simulink model "BSCU_Duration"  (Simulink 8.7)
settings: Solver=VariableStepAuto  StartTime=0.0  StopTime=10.0  RelTol=1e-3
settings Model: Creator=bourbouh  LastModifiedBy=bourbouh
settings DataIOCC: LimitDataPoints=off  SaveFormat=Dataset
settings DebuggingCC: UnderspecifiedInitializationDetection=Simplified  MergeDetectMultiDrivingBlocksExec=error
settings HardwareCC: ProdBitPerPointer=64  ProdLargestAtomicFloat=Float  ProdIntDivRoundTo=Zero  ProdEndianess=LittleEndian  ProdWordSize=64  ProdHWDeviceType=Intel->x86-64 (Windows64)
settings ModelReferenceCC: PropagateSignalLabelsOutOfModel=on
settings ConfigComp: CovModelRefEnable=off

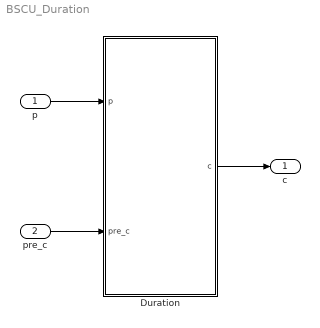
== system BSCU_Duration ==
  p : Inport
  pre_c : Inport  Port=2
  Duration : Stateflow chart  TreatAsAtomicUnit=on
  c : Outport
  wires:
  p/1 -> Duration/1(p)
  pre_c/1 -> Duration/2(pre_c)
  Duration/1(c) -> c/1

== stateflow chart Duration ==
  (default) -> (junction 6)
  (junction 6) -> (junction 7) [order 1] : [p]
  (junction 6) -> (junction 8) [order 2] : {c = 0;}
  (junction 7) -> (junction 9) : {c = pre_c+1;}
  (junction 9) -> (junction 8)
  (junction 8) -> (junction 10)
  data: p input boolean; c output int32; pre_c input int32
